simulink model "P5_3"  (R2020b)
settings: Solver=VariableStepAuto  StartTime=0.0  StopTime=inf  RelTol=1e-3
undefined symbols (not defined in the file): serial
libraries: instrumentlib x2
settings Model: Creator=escob  LastModifiedBy=Brizz

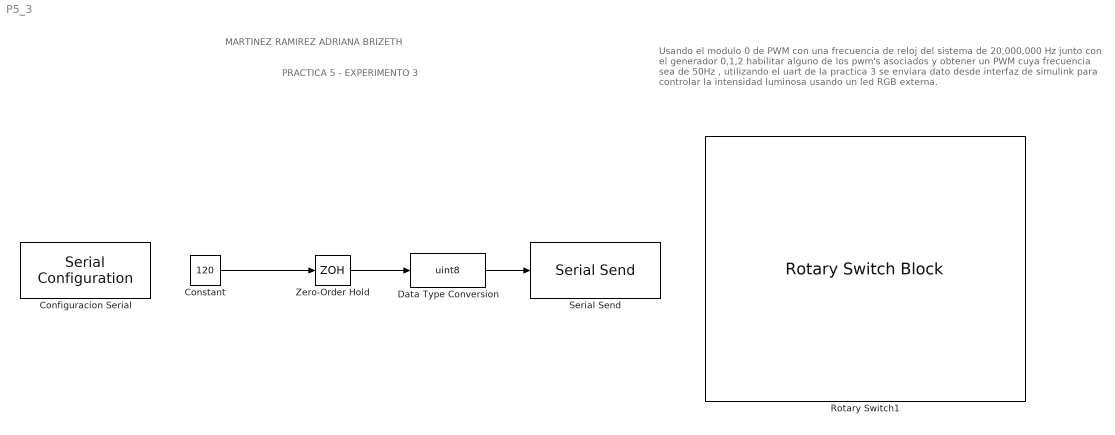
== system P5_3 ==
  note: Usando el modulo 0 de PWM con una frecuencia de reloj del sistema de 20,000,000 Hz junto con el generador 0,1,2 habilitar alguno de los pwm's asociados y obtener un PWM cuya frecuencia sea de 50Hz , utilizando el uart de la practica 3 se enviara dato desde interfaz de simulink para controlar la intensidad luminosa usando un led RGB externa.
  note: PRACTICA 5 - EXPERIMENTO 3
  note: MARTINEZ RAMIREZ ADRIANA BRIZETH
  Configuracion Serial : instrumentlib/Serial Configuration  Priority=-200000  ComPortMenu=COM4  ComPort=COM4  ObjConstructor=serial('COM4');  BaudRate=57600  DataBits=8  Parity=none  StopBits=1  FlowControl=none  Timeout=10  ByteOrder=LittleEndian
  Constant : Constant  Value=120
  "Data Type Conversion " : DataTypeConversion  OutDataTypeStr=uint8
  Rotary Switch1 : RotarySwitchBlock
      settings: Values={{'0%', '10%', '20%', '30%', '40%', '50%', '60%', '70%', '80%', '90%', '100%', '110%', '120%', '130%', '140%', '150%', '160%', '170%', '180%', '190%', '200%', '210%', '220%', '230%', '240%', '250%', '255%', 'R', 'G', 'B'}, [1 10 20 30 40 50 60 70 80 90 100 110 120 130 140 150 160 170 180 190 200 210 220 230 240 250 255 114 103 98]}
  Serial Send : instrumentlib/Serial Send  ComPortMenu=<Please select a port...>  ComPort=COM4  ObjConstructor=serial('COM4');  Terminator=<none>  EnableBlockingMode=on
  Zero-Order Hold : ZeroOrderHold  SampleTime=0.5
  wires:
  "Data Type Conversion "/1 -> Serial Send/1
  Zero-Order Hold/1 -> "Data Type Conversion "/1
  Constant/1 -> Zero-Order Hold/1
